simulink model "pPID"  (Simulink 9.2)
settings: Solver=ode45  StartTime=0  StopTime=10  MaxStep=0.02  RelTol=1e-3  AbsTol=1e-6
libraries: simulink x2
Description:
  | Inverted Pendulum with Animation
  | 
  | The animation is created using MATLAB(R) Handle Graphics(R).  The animation block is a masked
  | S-function.  For more information, use the context menu to look under the Animation block's mask
  | and open the S-function for editing.
settings Model: Creator=The MathWorks Inc.  LastModifiedBy=a  ExtModeAutoUpdateStatusClock=off
settings SolverCC: AutoScaleAbsTol=off
settings DataIOCC: ExternalInput=[]  InitialState=[]  LimitDataPoints=off  SaveOutput=off  SaveTime=off
settings OptimizationCC: BlockReduction=off  BooleanDataType=off  ExpressionDepthLimit=2147483647  InitFltsAndDblsToZero=on
settings DebuggingCC: SaveWithParameterizedLinksMsg=none  SignalResolutionControl=TryResolveAllWithWarning  MultiTaskDSMMsg=warning  MultiTaskCondExecSysMsg=none  SigSpecEnsureSampleTimeMsg=none
settings HardwareCC: TargetUnknown=on
settings GRTTargetCC: TargetFcnLib=ansi_tfl_tmw.mat

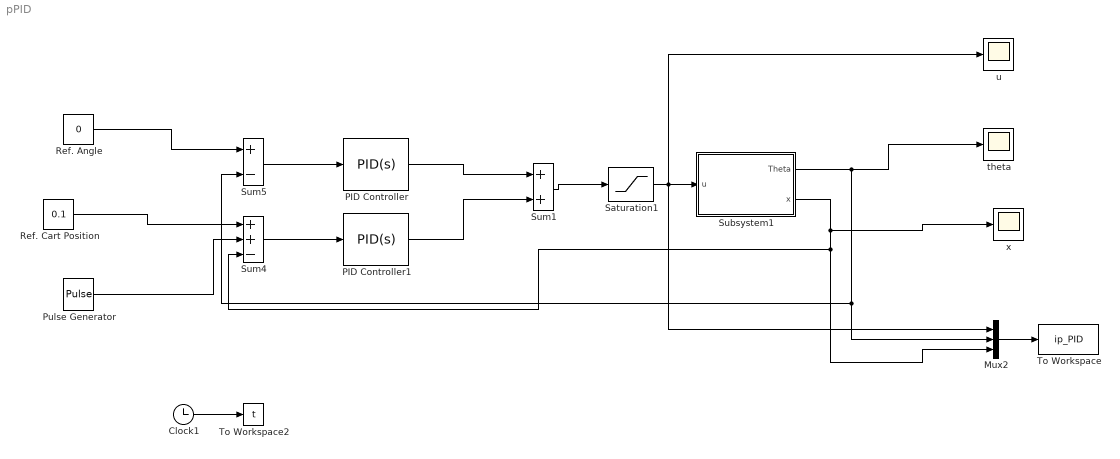
== system pPID ==
  Clock1 : Clock
  Mux2 : Mux  Inputs=3
  PID Controller : simulink/Continuous/PID Controller  Controller=PID  Form=Parallel  TimeDomain=Continuous-time  SampleTime=-1  IntegratorMethod=Forward Euler  FilterMethod=Forward Euler  ControllerParametersSource=internal  P=-40  I=0  D=-8  UseFilter=on  N=100  TunerSelectOption=Transfer Function Based (PID Tuner App)  InitialConditionSource=internal  InitialConditionForIntegrator=0  InitialConditionForFilter=0  DifferentiatorICPrevScaledInput=0  ExternalReset=none  TrackingMode=off  Kt=1  LimitOutput=off  UpperSaturationLimit=inf  LowerSaturationLimit=-inf  LinearizeAsGain=off  AntiWindupMode=none  Kb=1  POutMin=[]  POutMax=[]  IOutMin=[]  IOutMax=[]  DOutMin=[]  DOutMax=[]  NOutMin=[]  NOutMax=[]  SumOutMin=[]  SumOutMax=[]  SaturationOutMin=[]  SaturationOutMax=[]  PParamMin=[]  PParamMax=[]  IParamMin=[]  IParamMax=[]  DParamMin=[]  DParamMax=[]  NParamMin=[]  NParamMax=[]  KbParamMin=[]  KbParamMax=[]  KtParamMin=[]  KtParamMax=[]  KbOutMin=[]  KbOutMax=[]  KtOutMin=[]  KtOutMax=[]  IntegratorOutMin=[]  IntegratorOutMax=[]  FilterOutMin=[]  FilterOutMax=[]  SumI1OutMin=[]  SumI1OutMax=[]  SumI2OutMin=[]  SumI2OutMax=[]  SumI3OutMin=[]  SumI3OutMax=[]  SumI4OutMin=[]  SumI4OutMax=[]  SumDOutMin=[]  SumDOutMax=[]  DifferentiatorOutMin=[]  DifferentiatorOutMax=[]  FilterDiffOutCoefMin=[]  FilterDiffOutCoefMax=[]  ReciprocalOutMin=[]  ReciprocalOutMax=[]  SumDenOutMin=[]  SumDenOutMax=[]  SumNumOutMin=[]  SumNumOutMax=[]  DivideOutMin=[]  DivideOutMax=[]  IntegratorContinuousStateAttributes=''  IntegratorStateMustResolveToSignalObject=off  IntegratorRTWStateStorageClass=Auto  FilterContinuousStateAttributes=''  FilterStateMustResolveToSignalObject=off  FilterRTWStateStorageClass=Auto  ParallelPVariant=InternalParameters  IdealPVariant=Disabled  IVariant=InternalParameters  DVariant=InternalParameters  IntegratorVariant=Continuous  SatVariant=Disabled  AWVariant=Passthrough  PCopyVariant=Disabled  TRVariant=Disabled  FdbkBlocksVariant=Forward  IdealPFdbkVariant=Disabled  SatFdbkVariant=Disabled  DerivativeFilterVariant=ContFilter  NVariant=InternalParameters  NCopyVariant=Disabled  FilterICVariant=InternalICsFilter  IntegratorICVariant=InternalICs  ExternalResetVariant=Disabled  TRSumVariant=Passthrough  SumFdbkVariant=Disabled  SumVariant=Sum_PID
  PID Controller1 : simulink/Continuous/PID Controller  Controller=PID  Form=Parallel  TimeDomain=Continuous-time  SampleTime=-1  IntegratorMethod=Forward Euler  FilterMethod=Forward Euler  ControllerParametersSource=internal  P=-1  I=0  D=-3  UseFilter=on  N=100  TunerSelectOption=Transfer Function Based (PID Tuner App)  InitialConditionSource=internal  InitialConditionForIntegrator=0  InitialConditionForFilter=0  DifferentiatorICPrevScaledInput=0  ExternalReset=none  TrackingMode=off  Kt=1  LimitOutput=off  UpperSaturationLimit=inf  LowerSaturationLimit=-inf  LinearizeAsGain=off  AntiWindupMode=none  Kb=1  POutMin=[]  POutMax=[]  IOutMin=[]  IOutMax=[]  DOutMin=[]  DOutMax=[]  NOutMin=[]  NOutMax=[]  SumOutMin=[]  SumOutMax=[]  SaturationOutMin=[]  SaturationOutMax=[]  PParamMin=[]  PParamMax=[]  IParamMin=[]  IParamMax=[]  DParamMin=[]  DParamMax=[]  NParamMin=[]  NParamMax=[]  KbParamMin=[]  KbParamMax=[]  KtParamMin=[]  KtParamMax=[]  KbOutMin=[]  KbOutMax=[]  KtOutMin=[]  KtOutMax=[]  IntegratorOutMin=[]  IntegratorOutMax=[]  FilterOutMin=[]  FilterOutMax=[]  SumI1OutMin=[]  SumI1OutMax=[]  SumI2OutMin=[]  SumI2OutMax=[]  SumI3OutMin=[]  SumI3OutMax=[]  SumI4OutMin=[]  SumI4OutMax=[]  SumDOutMin=[]  SumDOutMax=[]  DifferentiatorOutMin=[]  DifferentiatorOutMax=[]  FilterDiffOutCoefMin=[]  FilterDiffOutCoefMax=[]  ReciprocalOutMin=[]  ReciprocalOutMax=[]  SumDenOutMin=[]  SumDenOutMax=[]  SumNumOutMin=[]  SumNumOutMax=[]  DivideOutMin=[]  DivideOutMax=[]  IntegratorContinuousStateAttributes=''  IntegratorStateMustResolveToSignalObject=off  IntegratorRTWStateStorageClass=Auto  FilterContinuousStateAttributes=''  FilterStateMustResolveToSignalObject=off  FilterRTWStateStorageClass=Auto  ParallelPVariant=InternalParameters  IdealPVariant=Disabled  IVariant=InternalParameters  DVariant=InternalParameters  IntegratorVariant=Continuous  SatVariant=Disabled  AWVariant=Passthrough  PCopyVariant=Disabled  TRVariant=Disabled  FdbkBlocksVariant=Forward  IdealPFdbkVariant=Disabled  SatFdbkVariant=Disabled  DerivativeFilterVariant=ContFilter  NVariant=InternalParameters  NCopyVariant=Disabled  FilterICVariant=InternalICsFilter  IntegratorICVariant=InternalICs  ExternalResetVariant=Disabled  TRSumVariant=Passthrough  SumFdbkVariant=Disabled  SumVariant=Sum_PID
  Pulse Generator : DiscretePulseGenerator  PulseType=Time based  Amplitude=0  Period=10  PulseWidth=5
  Ref. Angle : Constant  Value=0
  Ref. Cart Position : Constant  Value=0.1
  Saturation1 : Saturate  UpperLimit=100  LowerLimit=-100
  Subsystem1 : Subsystem
  Sum1 : Sum  SaturateOnIntegerOverflow=on  InputSameDT=on  OutDataTypeStr=Inherit: Same as first input
  Sum4 : Sum  Inputs=++-  SaturateOnIntegerOverflow=on  InputSameDT=on  OutDataTypeStr=Inherit: Same as first input
  Sum5 : Sum  Inputs=+-  SaturateOnIntegerOverflow=on  InputSameDT=on  OutDataTypeStr=Inherit: Same as first input
  To Workspace : ToWorkspace  VariableName=ip_PID  SampleTime=-1
  To Workspace2 : ToWorkspace  VariableName=t  SampleTime=-1
  theta : Scope
  u : Scope
  x : Scope
  wires:
  Sum1/1 -> Saturation1/1
  Saturation1/1 -> Mux2/1, Subsystem1/1(u), u/1
  Sum4/1 -> PID Controller1/1
  Sum5/1 -> PID Controller/1
  PID Controller/1 -> Sum1/1
  PID Controller1/1 -> Sum1/2
  Ref. Angle/1 -> Sum5/1
  Ref. Cart Position/1 -> Sum4/1
  Pulse Generator/1 -> Sum4/2
  Clock1/1 -> To Workspace2/1
  Mux2/1 -> To Workspace/1
  Subsystem1/1(Theta) -> Sum5/2, Mux2/2, theta/1
  Subsystem1/2(x) -> x/1, Sum4/3, Mux2/3

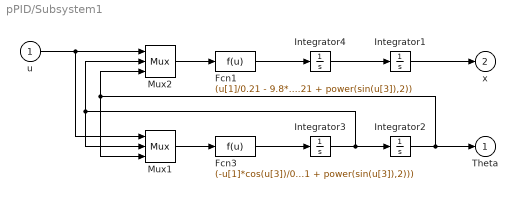
== system pPID/Subsystem1 ==
  u : Inport
  Fcn1 : Fcn  Expr=(u[1]/0.21 - 9.8*sin(u[3])*cos(u[3]) + (0.61/2)*power(u[2],2)*sin(u[3]))/(0.455/0.21 + power(sin(u[3]),2))
  Fcn3 : Fcn  Expr=(-u[1]*cos(u[3])/0.21 + (0.455+0.21)*9.8*sin(u[3])/0.21 - (0.61/2)*power(u[2],2)*sin(u[3])*cos(u[3]))/((0.61/2)*(0.455/0.21 + power(sin(u[3]),2)))
  Integrator{1..4} (4 alike) : Integrator
  Mux1 : Mux  Inputs=3
  Mux2 : Mux  Inputs=3
  Theta : Outport  InitialOutput=0
  x : Outport  Port=2  InitialOutput=0
  wires:
  Integrator1/1 -> x/1
  Fcn3/1 -> Integrator3/1
  Mux1/1 -> Fcn3/1
  Mux2/1 -> Fcn1/1
  Fcn1/1 -> Integrator4/1
  Integrator4/1 -> Integrator1/1
  u/1 -> Mux2/1, Mux1/1
  Integrator3/1 -> Integrator2/1, Mux2/2, Mux1/2
  Integrator2/1 -> Theta/1, Mux2/3, Mux1/3
